simulink model "DoubleSpin"  (R2023b)
settings: Solver=ode5  StartTime=0.0  StopTime=10.0  FixedStep=0.01  RelTol=1e-3
values from neighbouring files (symbols this model uses):
  I = diag(Iv)    [InitDoubleSpin.m]    (also in InitLab03.m)
  invI = inv(I)    [InitDoubleSpin.m]    (also in InitLab03.m)
  invJ = inv(J)    [InitDoubleSpin.m]
  J = diag(Jv)    [InitDoubleSpin.m]
  w0 = [1e-6; 0.005; 0.2]    [InitDoubleSpin.m]    (also in InitLab03.m = [2*pi; 0.5; 1])
  wr0 = 2*pi    (= 6.28318530718)    [InitDoubleSpin.m]
undefined symbols (not defined in the file or in its folder): Torque
libraries: matrix_library x4
settings Model: Creator=elisa  LastModifiedBy=elisa

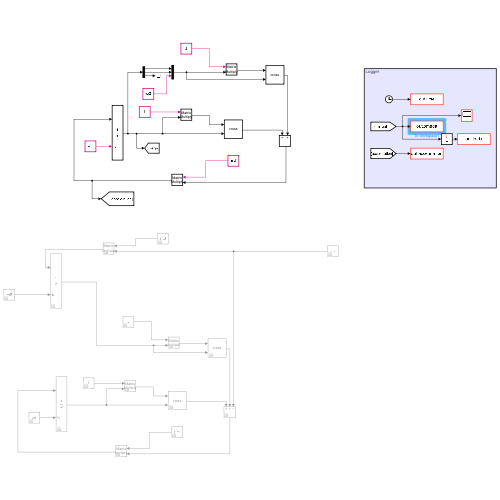
[thumbnail: Simulink's stored preview of the top-level diagram]
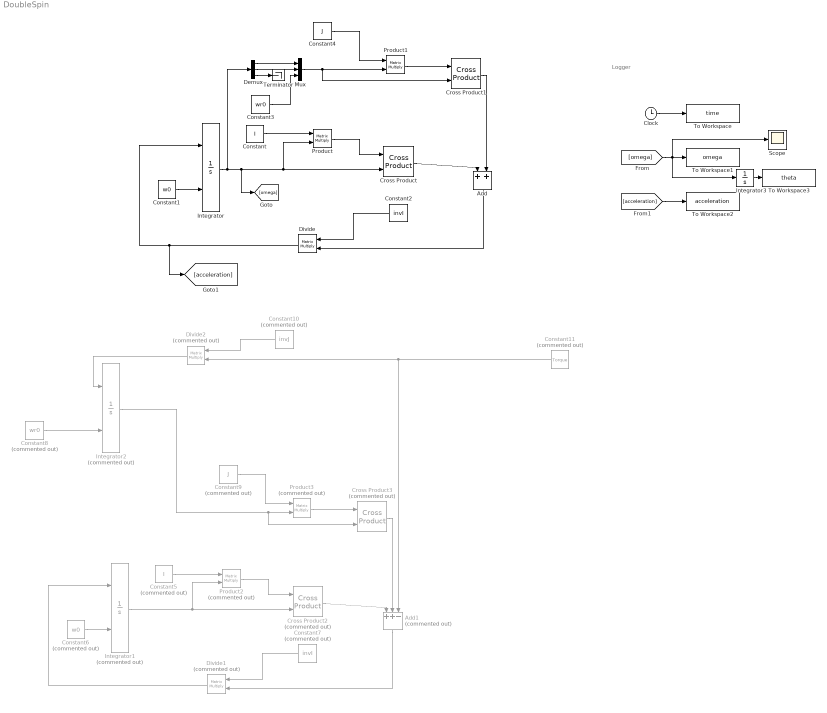
== system DoubleSpin ==
  note: Logger
  Add : Sum
  Add1 : Sum  Commented=on  Inputs=++-
  Clock : Clock
  Constant : Constant  Value=I
  Constant1 : Constant  Value=w0  VectorParams1D=off
  Constant10 : Constant  Commented=on  Value=invJ
  Constant11 : Constant  Commented=on  Value=Torque
  Constant2 : Constant  Value=invI
  Constant3 : Constant  Value=wr0
  Constant4 : Constant  Value=J
  Constant5 : Constant  Commented=on  Value=I
  Constant6 : Constant  Commented=on  Value=w0  VectorParams1D=off
  Constant7 : Constant  Commented=on  Value=invI
  Constant8 : Constant  Commented=on  Value=wr0
  Constant9 : Constant  Commented=on  Value=J
  Cross Product : matrix_library/Cross Product
  Cross Product1 : matrix_library/Cross Product
  Cross Product2 : matrix_library/Cross Product  Commented=on
  Cross Product3 : matrix_library/Cross Product  Commented=on
  Demux : Demux  Outputs=3
  Divide : Product  Inputs=**  Multiplication=Matrix(*)
  Divide1 : Product  Commented=on  Inputs=**  Multiplication=Matrix(*)
  Divide2 : Product  Commented=on  Inputs=**  Multiplication=Matrix(*)
  Integrator : Integrator  InitialConditionSource=external
  Integrator1 : Integrator  Commented=on  InitialConditionSource=external
  Integrator2 : Integrator  Commented=on  InitialConditionSource=external
  Integrator3 : Integrator
  Mux : Mux  Inputs=3
  Product : Product  Multiplication=Matrix(*)
  Product1 : Product  Multiplication=Matrix(*)
  Product2 : Product  Commented=on  Multiplication=Matrix(*)
  Product3 : Product  Commented=on  Multiplication=Matrix(*)
  Scope : Scope
  Terminator : Terminator
  To Workspace : ToWorkspace  VariableName=time  SaveFormat=Timeseries  SampleTime=-1
  To Workspace1 : ToWorkspace  VariableName=omega  SaveFormat=Timeseries  SampleTime=-1
  To Workspace2 : ToWorkspace  VariableName=acceleration  SaveFormat=Timeseries  SampleTime=-1
  To Workspace3 : ToWorkspace  VariableName=theta  SaveFormat=Timeseries  SampleTime=-1
  wires:
  Constant2/1 -> Divide/1
  Clock/1 -> To Workspace/1
  [acceleration] -> To Workspace2/1
  Constant1/1 -> Integrator/2
  Cross Product/1 -> Add/1
  Integrator/1 -> Demux/1, [omega], Product/2, Cross Product/2
  Constant/1 -> Product/1
  [omega] -> Integrator3/1, Scope/1, To Workspace1/1
  Divide/1 -> [acceleration], Integrator/1
  Product/1 -> Cross Product/1
  Product1/1 -> Cross Product1/1
  Constant4/1 -> Product1/1
  Add/1 -> Divide/2
  Cross Product1/1 -> Add/2
  Cross Product2/1 -> Add1/1
  Add1/1 -> Divide1/2
  Product2/1 -> Cross Product2/1
  Constant5/1 -> Product2/1
  Integrator1/1 -> Product2/2, Cross Product2/2
  Constant6/1 -> Integrator1/2
  Constant7/1 -> Divide1/1
  Divide1/1 -> Integrator1/1
  Cross Product3/1 -> Add1/2
  Product3/1 -> Cross Product3/1
  Constant9/1 -> Product3/1
  Integrator2/1 -> Cross Product3/2, Product3/2
  Constant8/1 -> Integrator2/2
  Constant10/1 -> Divide2/1
  Divide2/1 -> Integrator2/1
  Constant11/1 -> Add1/3, Divide2/2
  Demux/3 -> Terminator/1
  Demux/2 -> Mux/2
  Demux/1 -> Mux/1
  Constant3/1 -> Mux/3
  Mux/1 -> Product1/2, Cross Product1/2
  Integrator3/1 -> To Workspace3/1
